simulink model "controlPID"  (R2019a)
settings: Solver=VariableStepAuto  StartTime=0.0  StopTime=20  RelTol=1e-3
libraries: simulink x1
settings Model: Creator=WALTER  LastModifiedBy=WALTER

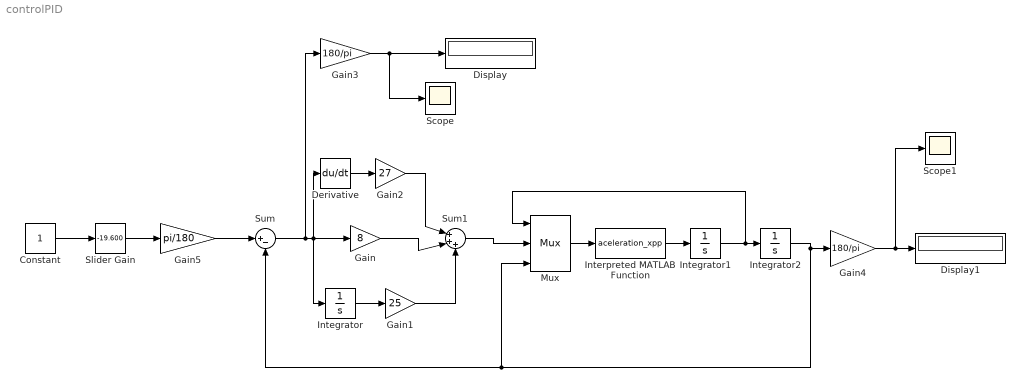
== system controlPID ==
  Constant : Constant
  Derivative : Derivative
  Display : Display
  Display1 : Display
  Gain : Gain  Gain=8
  Gain1 : Gain  Gain=25
  Gain2 : Gain  Gain=27
  Gain3 : Gain  Gain=180/pi
  Gain4 : Gain  Gain=180/pi
  Gain5 : Gain  Gain=pi/180
  Integrator : Integrator
  Integrator1 : Integrator
  Integrator2 : Integrator
  Interpreted MATLAB Function : MATLABFcn  MATLABFcn=aceleration_xpp
  Mux : Mux  Inputs=3
      settings: DisplayOption=signals
  Scope : Scope
  Scope1 : Scope
  Slider Gain : simulink/Math Operations/Slider Gain  gain=-19.600  low=-20  high=20
  Sum : Sum  Inputs=|+-
  Sum1 : Sum  Inputs=|+++
  wires:
  Sum1/1 -> Mux/2
  Sum/1 -> Gain3/1, Integrator/1, Gain/1, Derivative/1
  Derivative/1 -> Gain2/1
  Gain2/1 -> Sum1/1
  Gain/1 -> Sum1/2
  Gain1/1 -> Sum1/3
  Integrator/1 -> Gain1/1
  Slider Gain/1 -> Gain5/1
  Constant/1 -> Slider Gain/1
  Gain3/1 -> Scope/1, Display/1
  Integrator1/1 -> Mux/1, Integrator2/1
  Integrator2/1 -> Gain4/1, Mux/3, Sum/2
  Gain4/1 -> Scope1/1, Display1/1
  Mux/1 -> Interpreted MATLAB Function/1
  Interpreted MATLAB Function/1 -> Integrator1/1
  Gain5/1 -> Sum/1
